simulink model "tractor_plant"  (R2024b)
settings: Solver=ode4  StartTime=0.0  StopTime=tStop  FixedStep=0.01  RelTol=1e-3
model workspace (MAT data in the model file):
  imuXRearAxleM = 0
  p0 = [10178.6; 1.6562; 1.1538; 19450.5265478; 356356.4449; 270000; 1.10369051]
  p1 = [10178.6; 1.6562; 1.1538; 19450.5265478; 356356.4449; 270000; 1.10369051]
  tEnd = 0
  tStart = 0
  tStop = 10
  x0_plant = [0; 0; 0; 0; 0; 0]
settings Model: Creator=Jhuessy  LastModifiedBy=Jhuessy
settings DataIOCC: SaveFormat=Array

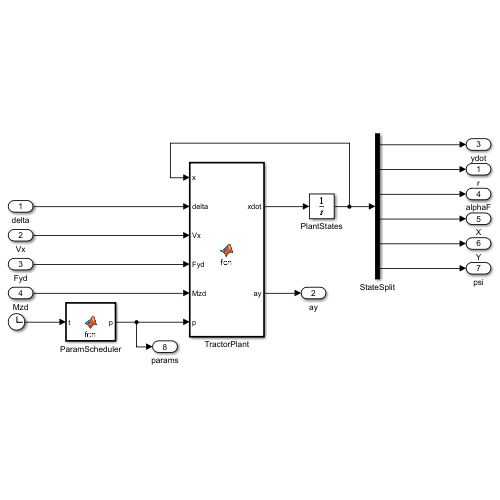
[thumbnail: Simulink's stored preview of the top-level diagram]
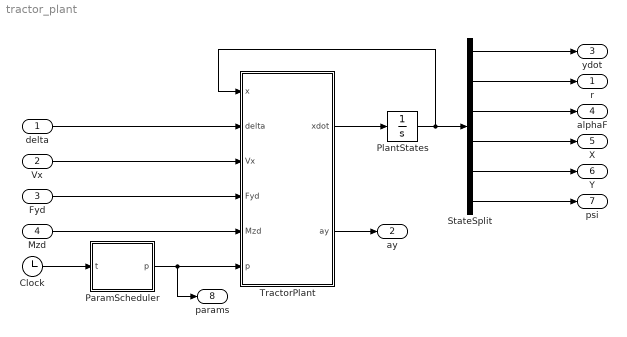
== system tractor_plant ==
  delta : Inport
  Vx : Inport  Port=2
  Fyd : Inport  Port=3
  Mzd : Inport  Port=4
  Clock : Clock
  ParamScheduler : MATLAB Function  TreatAsAtomicUnit=on
  PlantStates : Integrator  InitialCondition=x0_plant
  StateSplit : Demux  Outputs=6
  TractorPlant : MATLAB Function  TreatAsAtomicUnit=on
  r : Outport
  ay : Outport  Port=2
  ydot : Outport  Port=3
  alphaF : Outport  Port=4
  X : Outport  Port=5
  Y : Outport  Port=6
  psi : Outport  Port=7
  params : Outport  Port=8
  wires:
  Clock/1 -> ParamScheduler/1(t)
  ParamScheduler/1(p) -> params/1, TractorPlant/6(p)
  PlantStates/1 -> TractorPlant/1(x), StateSplit/1
  delta/1 -> TractorPlant/2(delta)
  Vx/1 -> TractorPlant/3(Vx)
  Fyd/1 -> TractorPlant/4(Fyd)
  Mzd/1 -> TractorPlant/5(Mzd)
  TractorPlant/1(xdot) -> PlantStates/1
  TractorPlant/2(ay) -> ay/1
  StateSplit/1 -> ydot/1
  StateSplit/2 -> r/1
  StateSplit/3 -> alphaF/1
  StateSplit/4 -> X/1
  StateSplit/5 -> Y/1
  StateSplit/6 -> psi/1

== matlab function tractor_plant/TractorPlant ==
  data: x input; xdot output size=6; delta input; Vx input; Fyd input; Mzd input; p input; ay output; imuXRearAxleM parameter
function [xdot, ay] = fcn(x, delta, Vx, Fyd, Mzd, p, imuXRearAxleM)

% x = [ydot; r; alphaF; X; Y; psi], p = [m lf lr Izz Caf Car sigmaF]
m = p(1); lf = p(2); lr = p(3); Izz = p(4); Caf = p(5); Car = p(6); sig = p(7);

v = x(1); r = x(2); af = x(3); psi = x(6);

Fyf = Caf*af;
Fyr = -Car*(v - lr*r)/Vx;

vdot = (Fyf + Fyr + Fyd)/m - Vx*r;
rdot = (lf*Fyf - lr*Fyr + Mzd)/Izz;
afdot = (Vx*delta - v - lf*r - Vx*af)/sig;
xdot = [vdot; rdot; afdot; Vx*cos(psi) - v*sin(psi); Vx*sin(psi) + v*cos(psi); r];

% IMU is fixed to the chassis at imuXRearAxleM ahead of the rear axle, i.e. (imuXRearAxleM - lr) ahead of the CG
ay = vdot + Vx*r + (imuXRearAxleM - lr)*rdot;

== matlab function tractor_plant/ParamScheduler ==
  data: t input; p output size=7; p0 parameter; p1 parameter; tStart parameter; tEnd parameter
function p = fcn(t, p0, p1, tStart, tEnd)
% Blend nominal parameters p0 into p1 between tStart and tEnd (step if tEnd ~ tStart).
% p = [m lf lr Izz Caf Car sigmaF]
s = min(max((t - tStart)/max(tEnd - tStart, 1e-6), 0), 1);
p = p0 + s*(p1 - p0);
